simulink model "dumbxxx"  (R2015a)
settings: Solver=FixedStepDiscrete  SolverMode=SingleTasking  StartTime=0.0  StopTime=10.0  FixedStep=T0  RelTol=1e-3  AbsTol=1e-6
InitFcn:
  | T0=0.003;
libraries: simulink_extras x1
Description:
  | The van der Pol Equation
  | 
  | This is a simulation of a nonlinear second order system.
settings Model: SimulationMode=external  CovSFcnEnable=off  ExtModeTrigDuration=100000  ExtModeAutoUpdateStatusClock=off  Creator=The MathWorks Inc.  LastModifiedBy=RBoth
settings DataIOCC: ExternalInput=[]  InitialState=[]  LimitDataPoints=off  SignalLoggingSaveFormat=ModelDataLogs  SaveOutput=off  SignalLogging=off  DSMLogging=off  SaveTime=off
settings OptimizationCC: BlockReduction=off  BooleanDataType=off  ExpressionDepthLimit=2147483647  InitFltsAndDblsToZero=on  BufferReusableBoundary=off
settings DebuggingCC: SaveWithParameterizedLinksMsg=none  UnderspecifiedInitializationDetection=Classic  MergeDetectMultiDrivingBlocksExec=none  SignalResolutionControl=TryResolveAllWithWarning  MultiTaskDSMMsg=warning  MultiTaskCondExecSysMsg=none  FcnCallInpInsideContextMsg=UseLocalSettings  BusObjectLabelMismatch=none  StateNameClashWarn=warning
settings HardwareCC: TargetLongLongMode=on  TargetIntDivRoundTo=Zero  TargetEndianess=LittleEndian  TargetHWDeviceType=MATLAB Host  ProdEqTarget=off
settings SFSimCC: SimParseCustomCode=off
settings RTWCC: SystemTargetFile=grt_panda.tlc  TemplateMakefile=grt_panda.tmf  Description=Panda Board Real-Time Target
settings GRTTargetCC: ExtMode=on  ExtModeMexArgs='10.0.0.1', 1

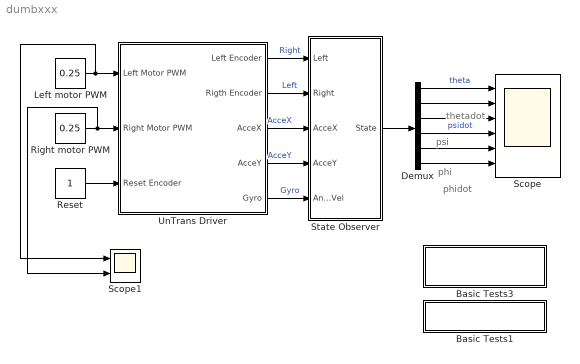
== system dumbxxx ==
  note: thetadot
  note: psi
  note: phi
  note: phidot
  Basic Tests1 : Subsystem
      settings: OpenFcn=|
      | UnTransTCPStart('10.0.0.1',20004)
      | fprintf('\nActivated\n')
      mask Display: fprintf( 'Activate Target' )
  Basic Tests3 : Subsystem
      settings: OpenFcn=|
      | UnTransTCPStop('10.0.0.1',20004);
      | MODEL_NAME = gcs;
      | slbuild(MODEL_NAME)
      | cd([MODEL_NAME '_grt_rtw'])
      | PSCP = ['!' matlabroot '\toolbox\UnTrans\tools\pscp'];
      | eval([PSCP ' -pw panda ' MODEL_NAME ' panda@10.0.0.1:/home/panda/inteco/rt_model'])
      | cd('..')
      | fprintf('\nReady to activate\n')
      mask Display: fprintf( 'Build & Send\nto Target' )
  Demux : Demux  Outputs=6
  Left motor PWM : Constant  Value=0.25
  Reset : Constant
  Right motor PWM : Constant  Value=0.25
  Scope : Scope  NumInputPorts=6
      settings: YMin=-5~-5~-5~-5~-5~-5  YMax=5~5~5~5~5~5  SaveName=ScopeData025out
  Scope1 : Scope  NumInputPorts=2
      settings: YMin=-5~-5  YMax=5~5  SaveName=ScopeData025in
  State Observer : Subsystem
  UnTrans Driver : Subsystem  mask{T0=T0}
      mask prompts: T0 "Sampling Period:"
      mask Display: image(imread('intebot_small2.bmp'))
  wires:
  Reset/1 -> UnTrans Driver/3(Reset Encoder)
  Right motor PWM/1 -> Scope1/2, UnTrans Driver/2(Right Motor PWM)
  Left motor PWM/1 -> Scope1/1, UnTrans Driver/1(Left Motor PWM)
  State Observer/1(State) -> Demux/1
  Demux/1 -> Scope/1  "theta"
  Demux/2 -> Scope/2
  Demux/3 -> Scope/3
  Demux/4 -> Scope/4  "psidot"
  Demux/5 -> Scope/5
  Demux/6 -> Scope/6
  UnTrans Driver/2(Rigth Encoder) -> State Observer/2(Right)  "Left"
  UnTrans Driver/3(AcceX) -> State Observer/3(AcceX)  "AcceX"
  UnTrans Driver/1(Left Encoder) -> State Observer/1(Left)  "Right"
  UnTrans Driver/4(AcceY) -> State Observer/4(AcceY)  "AcceY"
  UnTrans Driver/5(Gyro) -> State Observer/5(AngleVel)  "Gyro"

== system dumbxxx/Basic Tests1 ==

== system dumbxxx/Basic Tests3 ==

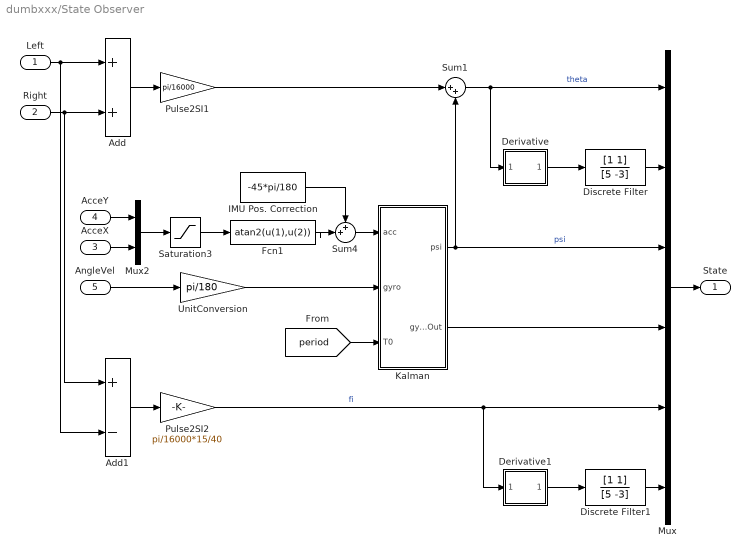
== system dumbxxx/State Observer ==
  Left : Inport
  Right : Inport  Port=2
  AcceX : Inport  Port=3
  AcceY : Inport  Port=4
  AngleVel : Inport  Port=5
  Add : Sum
  Add1 : Sum  Inputs=+-
  Derivative : Subsystem
  Derivative1 : Subsystem
  Discrete Filter : DiscreteFilter  Numerator=[1 1]  Denominator=[5 -3]
  Discrete Filter1 : DiscreteFilter  Numerator=[1 1]  Denominator=[5 -3]
  Fcn1 : Fcn  Expr=atan2(u(1),u(2))
  IMU Pos. Correction : Constant  Value=-45*pi/180
  Kalman : MATLAB Function  TreatAsAtomicUnit=on
  Mux : Mux  Inputs=6
  Mux2 : Mux  Inputs=2
  Pulse2SI1 : Gain  Gain=pi/16000
  Pulse2SI2 : Gain  Gain=pi/16000*15/40
  Saturation3 : Saturate  UpperLimit=1  LowerLimit=0
  Sum1 : Sum  Inputs=|++
  Sum4 : Sum  Inputs=++|
  UnitConversion : Gain  Gain=pi/180
  State : Outport
  wires:
  AngleVel/1 -> UnitConversion/1
  Mux2/1 -> Saturation3/1
  Mux/1 -> State/1
  Sum4/1 -> Kalman/1(acc)
  IMU Pos. Correction/1 -> Sum4/1
  UnitConversion/1 -> Kalman/2(gyro)
  AcceX/1 -> Mux2/2
  AcceY/1 -> Mux2/1
  Saturation3/1 -> Fcn1/1
  Fcn1/1 -> Sum4/2
  [period] -> Kalman/3(T0)
  Derivative/1(Vel) -> Discrete Filter/1
  Right/1 -> Add/2, Add1/1
  Add/1 -> Pulse2SI1/1
  Left/1 -> Add/1, Add1/2
  Add1/1 -> Pulse2SI2/1
  Derivative1/1(Vel) -> Discrete Filter1/1
  Pulse2SI2/1 -> Mux/5, Derivative1/1(Pos)  "fi"
  Discrete Filter1/1 -> Mux/6
  Kalman/1(psi) -> Sum1/2, Mux/3  "psi"
  Kalman/2(gyroOut) -> Mux/4
  Discrete Filter/1 -> Mux/2
  Pulse2SI1/1 -> Sum1/1
  Sum1/1 -> Mux/1, Derivative/1(Pos)  "theta"

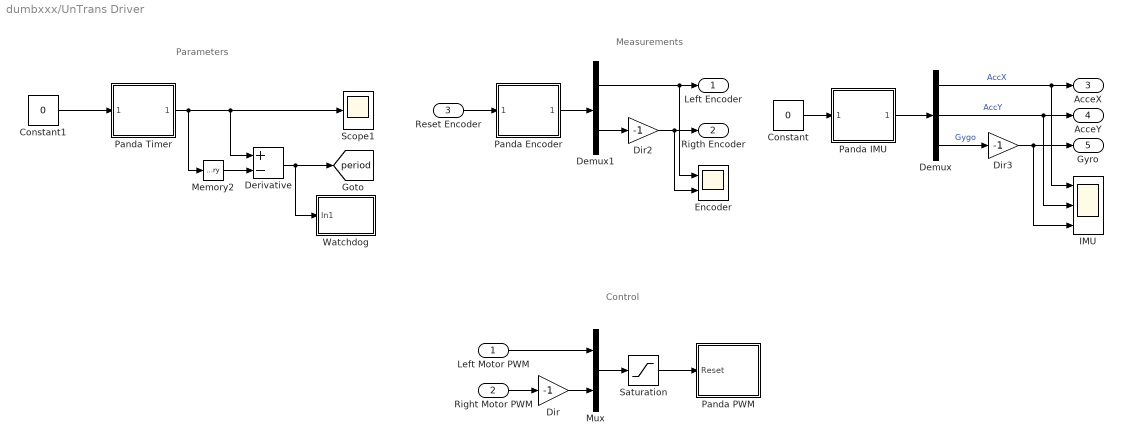
== system dumbxxx/UnTrans Driver ==
  note: Control
  note: Measurements
  note: Parameters
  Left Motor PWM : Inport
  Right Motor PWM : Inport  Port=2
  Reset Encoder : Inport  Port=3
  Constant : Constant  Value=0
  Constant1 : Constant  Value=0
  Demux : Demux  Outputs=3
  Demux1 : Demux  Outputs=2
  Derivative : Sum  Inputs=+-
  Dir : Gain  Gain=-1  SaturateOnIntegerOverflow=on  OutDataTypeStr=Inherit: Same as input  ParamDataTypeStr=Inherit: Same as input
  Dir2 : Gain  Gain=-1  SaturateOnIntegerOverflow=on  OutDataTypeStr=Inherit: Same as input  ParamDataTypeStr=Inherit: Same as input
  Dir3 : Gain  Gain=-1  SaturateOnIntegerOverflow=on  OutDataTypeStr=Inherit: Same as input  ParamDataTypeStr=Inherit: Same as input
  Encoder : Scope  NumInputPorts=2
      settings: TimeRange=45  YMin=0~375  YMax=37500~700  SaveName=encoder_RT  MaxDataPoints=120
  IMU : Scope  NumInputPorts=3
      settings: TimeRange=30  YMin=0.13~0.986~-1.5  YMax=0.146~1.001~0.7  SaveName=imu_RT  MaxDataPoints=120
  Memory2 : Memory
  Mux : Mux  Inputs=2
  Panda Encoder : Subsystem  mask(Timer){T0=T0}
      mask prompts: T0 "Sample Time (sec):"
      mask help: RT-DAC PCI Device Driver
      mask Help: Set up each field for your specific hardware configuration.
      mask Display: plot(0,0,100,100,[90,80,80,11,11],[90,90,20,20,80],[11,80],[80,80],[80,80],[20,14],[80,85,85,80],[45,45,66,66],[45,45,74,74],[20,13,13,20],[15,27,27,15,15],[75,75,26,26,75],[33,48,48,33,33],[75,75,55,55,75],[55,55,71,71,55],[55,75,75,55,55],[33,41,41,33,33],[50,50,27,27,50],[48,56,56,48,48],[50,50,27,27,50],[62,70,70,62,62],[50,50,27,27,50])
  Panda IMU : Subsystem  mask(Timer){T0=T0}
      mask prompts: T0 "Sample Time (sec):"
      mask help: RT-DAC PCI Device Driver
      mask Help: Set up each field for your specific hardware configuration.
      mask Display: plot(0,0,100,100,[90,80,80,11,11],[90,90,20,20,80],[11,80],[80,80],[80,80],[20,14],[80,85,85,80],[45,45,66,66],[45,45,74,74],[20,13,13,20],[15,27,27,15,15],[75,75,26,26,75],[33,48,48,33,33],[75,75,55,55,75],[55,55,71,71,55],[55,75,75,55,55],[33,41,41,33,33],[50,50,27,27,50],[48,56,56,48,48],[50,50,27,27,50],[62,70,70,62,62],[50,50,27,27,50])
  Panda PWM : Subsystem  mask(Timer){T0=T0}
      mask prompts: T0 "Sample Time (sec):"
      mask help: RT-DAC PCI Device Driver
      mask Help: Set up each field for your specific hardware configuration.
      mask Display: plot(0,0,100,100,[90,80,80,11,11],[90,90,20,20,80],[11,80],[80,80],[80,80],[20,14],[80,85,85,80],[45,45,66,66],[45,45,74,74],[20,13,13,20],[15,27,27,15,15],[75,75,26,26,75],[33,48,48,33,33],[75,75,55,55,75],[55,55,71,71,55],[55,75,75,55,55],[33,41,41,33,33],[50,50,27,27,50],[48,56,56,48,48],[50,50,27,27,50],[62,70,70,62,62],[50,50,27,27,50])
  "Panda Timer " : Subsystem  mask(Timer){T0=T0}
      mask prompts: T0 "Sample Time (sec):"
      mask help: RT-DAC PCI Device Driver
      mask Help: Set up each field for your specific hardware configuration.
      mask Display: plot(0,0,100,100,[90,80,80,11,11],[90,90,20,20,80],[11,80],[80,80],[80,80],[20,14],[80,85,85,80],[45,45,66,66],[45,45,74,74],[20,13,13,20],[15,27,27,15,15],[75,75,26,26,75],[33,48,48,33,33],[75,75,55,55,75],[55,55,71,71,55],[55,75,75,55,55],[33,41,41,33,33],[50,50,27,27,50],[48,56,56,48,48],[50,50,27,27,50],[62,70,70,62,62],[50,50,27,27,50])
  Saturation : Saturate  UpperLimit=1  LowerLimit=-1
  Scope1 : Scope
      settings: TickLabels=on  TimeRange=20  YMin=1.35987e+09  YMax=1.50301e+09  SaveName=timer_RT
  Watchdog : Subsystem
  Left Encoder : Outport  InitialOutput=0
  Rigth Encoder : Outport  Port=2  InitialOutput=0
  AcceX : Outport  Port=3  InitialOutput=0
  AcceY : Outport  Port=4  InitialOutput=0
  Gyro : Outport  Port=5  InitialOutput=0
  tag scope: period=global
  wires:
  Mux/1 -> Saturation/1
  Right Motor PWM/1 -> Dir/1
  Demux1/2 -> Dir2/1
  Panda Encoder/1(Timer) -> Demux1/1
  Reset Encoder/1 -> Panda Encoder/1(Reset)
  Dir2/1 -> Encoder/2, Rigth Encoder/1
  Demux1/1 -> Encoder/1, Left Encoder/1
  Panda IMU/1(Timer) -> Demux/1
  Demux/1 -> AcceX/1, IMU/1  "AccX"
  Demux/2 -> AcceY/1, IMU/2  "AccY"
  Demux/3 -> Dir3/1  "Gygo"
  "Panda Timer "/1(Timer) -> Memory2/1, Scope1/1, Derivative/1
  Saturation/1 -> Panda PWM/1(Reset)
  Memory2/1 -> Derivative/2
  Derivative/1 -> [period], Watchdog/1(In1)
  Constant/1 -> Panda IMU/1(Reset)
  Constant1/1 -> "Panda Timer "/1(Reset)
  Dir/1 -> Mux/2
  Left Motor PWM/1 -> Mux/1
  Dir3/1 -> Gyro/1, IMU/3

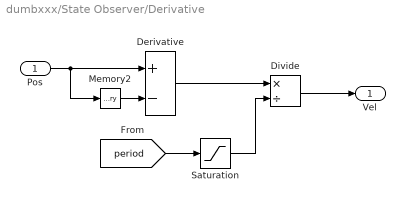
== system dumbxxx/State Observer/Derivative ==
  Pos : Inport
  Derivative : Sum  Inputs=+-
  Divide : Product  Inputs=*/
  Memory2 : Memory
  Saturation : Saturate  UpperLimit=1  LowerLimit=0.001
  Vel : Outport
  wires:
  [period] -> Saturation/1
  Memory2/1 -> Derivative/2
  Pos/1 -> Memory2/1, Derivative/1
  Derivative/1 -> Divide/1
  Saturation/1 -> Divide/2
  Divide/1 -> Vel/1

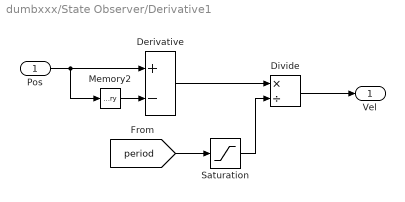
== system dumbxxx/State Observer/Derivative1 ==
  Pos : Inport
  Derivative : Sum  Inputs=+-
  Divide : Product  Inputs=*/
  Memory2 : Memory
  Saturation : Saturate  UpperLimit=1  LowerLimit=0.001
  Vel : Outport
  wires:
  [period] -> Saturation/1
  Memory2/1 -> Derivative/2
  Pos/1 -> Memory2/1, Derivative/1
  Derivative/1 -> Divide/1
  Saturation/1 -> Divide/2
  Divide/1 -> Vel/1

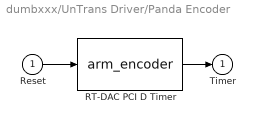
== system dumbxxx/UnTrans Driver/Panda Encoder ==
  Reset : Inport
  RT-DAC PCI D Timer : S-Function  FunctionName=arm_encoder  Parameters=T0
  Timer : Outport  InitialOutput=0
  wires:
  RT-DAC PCI D Timer/1 -> Timer/1
  Reset/1 -> RT-DAC PCI D Timer/1

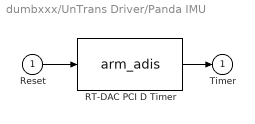
== system dumbxxx/UnTrans Driver/Panda IMU ==
  Reset : Inport
  RT-DAC PCI D Timer : S-Function  FunctionName=arm_adis  Parameters=T0
  Timer : Outport  InitialOutput=0
  wires:
  Reset/1 -> RT-DAC PCI D Timer/1
  RT-DAC PCI D Timer/1 -> Timer/1

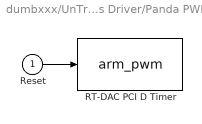
== system dumbxxx/UnTrans Driver/Panda PWM ==
  Reset : Inport
  RT-DAC PCI D Timer : S-Function  FunctionName=arm_pwm  Parameters=T0
  wires:
  Reset/1 -> RT-DAC PCI D Timer/1

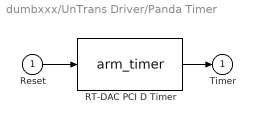
== system dumbxxx/UnTrans Driver/Panda Timer  ==
  Reset : Inport
  RT-DAC PCI D Timer : S-Function  FunctionName=arm_timer  Parameters=T0
  Timer : Outport  InitialOutput=0
  wires:
  RT-DAC PCI D Timer/1 -> Timer/1
  Reset/1 -> RT-DAC PCI D Timer/1

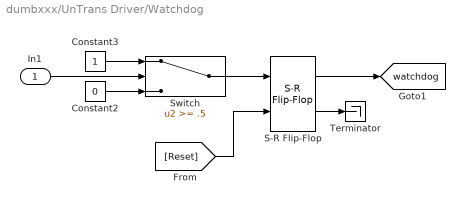
== system dumbxxx/UnTrans Driver/Watchdog ==
  In1 : Inport
  Constant2 : Constant  Value=0
  Constant3 : Constant
  S-R Flip-Flop : simulink_extras/Flip Flops/S-R Flip-Flop  initial_condition=0
  Switch : Switch  Threshold=.5
  Terminator : Terminator
  tag scope: watchdog=global
  wires:
  Constant3/1 -> Switch/1
  Constant2/1 -> Switch/3
  In1/1 -> Switch/2
  Switch/1 -> S-R Flip-Flop/1
  S-R Flip-Flop/1 -> [watchdog]
  S-R Flip-Flop/2 -> Terminator/1
  [Reset] -> S-R Flip-Flop/2

== matlab function dumbxxx/State Observer/Kalman ==
  data: acc input; gyro input; psi output; gyroOut output; T0 input
function [psi,gyroOut] = fcn(acc, gyro, T0)
%#codegen
persistent A B H Q R P I x_est

if isempty(P)
    H = [1 0 0];
    Q = [1   0       0;
         0      0.001    0;
         0      0       0.01];
    R = 1e6;
    x_est = [acc; 0; gyro];
    P = eye(3)*0.5;
    I = eye(3);
end

dt = T0;
if dt < .002 
    dt = .002;
elseif dt > .01
    dt = .01;
end
    
A = [1 0 -dt; 0 0 -1; 0 0 1];
B = [dt; 1; 0];

%time update (prediction)
x_est = A*x_est + B*gyro;
P = A*P*A' + Q;

%measurement update (correction)
K = P*H'/(H*P*H'+R);
x_est = x_est + K*(acc - H*x_est);
P = (I - K*H)*P;

psi = H*x_est;
gyroOut=x_est(2);
